simulink model "RTR_2st"  (R2020a)
settings: Solver=ode45  StartTime=0.0  StopTime=T  RelTol=1e-8
values from neighbouring files (symbols this model uses):
  g = 9.81    [TestingIkRTR.m]    (also in TestingScript.m; TestingScriptRTR.m)
  Kd1 = Kp1/10    (= 100)    [TestingIkRTR.m]    (also in TestingScript.m; TestingScriptRTR.m)
  Kp1 = 1000    [TestingIkRTR.m]    (also in TestingScript.m; TestingScriptRTR.m)
  l2 = 0.3    [TestingIkRTR.m]    (also in TestingScriptRTR.m)
  l3 = 0.2    [TestingIkRTR.m]    (also in TestingScriptRTR.m)
  m2 = 20    [TestingIkRTR.m]    (also in TestingScriptRTR.m)
  m3 = 20    [TestingIkRTR.m]    (also in TestingScriptRTR.m)
  O4 = 0.77    [TestingScript.m]
settings Model: Creator=ja  LastModifiedBy=ja

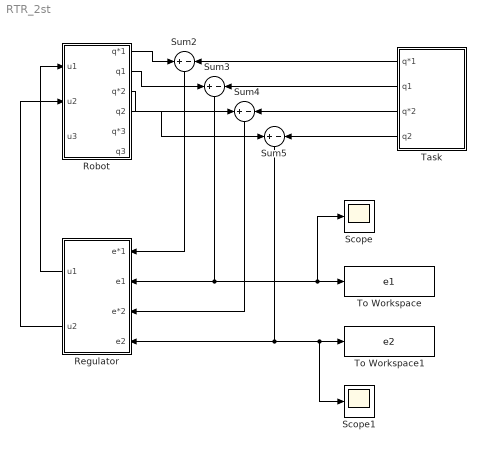
== system RTR_2st ==
  Regulator : Subsystem
  Robot : Subsystem
  Scope : Scope
  Scope1 : Scope
  Sum{2..5} (4 alike) : Sum  Inputs=+-
  Task : Subsystem
  To Workspace : ToWorkspace  VariableName=e1  SampleTime=-1
  To Workspace1 : ToWorkspace  VariableName=e2  SampleTime=-1
  wires:
  Sum4/1 -> Regulator/3(e*2)
  Sum3/1 -> Regulator/2(e1), Scope/1, To Workspace/1
  Sum2/1 -> Regulator/1(e*1)
  Robot/3(q*2) -> Sum4/1
  Robot/4(q2) -> Sum5/1
  Task/1(q*1) -> Sum2/2
  Sum5/1 -> Regulator/4(e2), Scope1/1, To Workspace1/1
  Robot/2(q1) -> Sum3/1
  Task/2(q1) -> Sum3/2
  Regulator/1(" u1") -> Robot/1(u1)
  Task/4(q2) -> Sum5/2
  Regulator/2(u2) -> Robot/2(u2)
  Robot/1(q*1) -> Sum2/1
  Task/3(q*2) -> Sum4/2

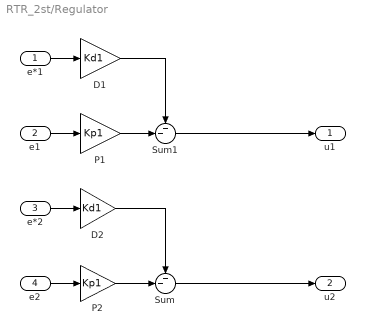
== system RTR_2st/Regulator ==
  e*1 : Inport
  e1 : Inport  Port=2
  e*2 : Inport  Port=3
  e2 : Inport  Port=4
  D1 : Gain  Gain=Kd1
  D2 : Gain  Gain=Kd1
  P1 : Gain  Gain=Kp1
  P2 : Gain  Gain=Kp1
  Sum : Sum  Inputs=--|
  Sum1 : Sum  Inputs=--|
  " u1" : Outport
  u2 : Outport  Port=2
  wires:
  e2/1 -> P2/1
  Sum/1 -> u2/1
  e*2/1 -> D2/1
  e1/1 -> P1/1
  Sum1/1 -> " u1"/1
  e*1/1 -> D1/1
  D1/1 -> Sum1/1
  P1/1 -> Sum1/2
  D2/1 -> Sum/1
  P2/1 -> Sum/2

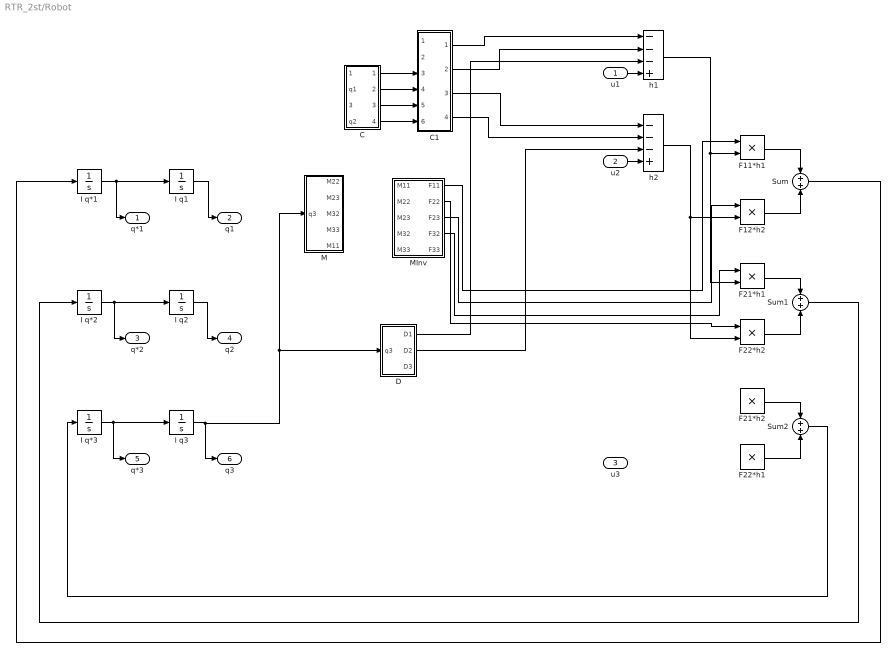
== system RTR_2st/Robot ==
  u1 : Inport
  u2 : Inport  Port=2
  u3 : Inport  Port=3
  C : Subsystem
  C1 : Subsystem
  D : Subsystem
  F11*h1 : Product
  F12*h2 : Product
  F21*h1 : Product
  F21*h2 : Product
  F22*h1 : Product
  F22*h2 : Product
  I q*1 : Integrator
  I q*2 : Integrator
  I q*3 : Integrator
  I q1 : Integrator
  I q2 : Integrator
  I q3 : Integrator
  M : Subsystem
  MInv : MATLAB Function  TreatAsAtomicUnit=on
  Sum : Sum
  Sum1 : Sum
  Sum2 : Sum
  h1 : Sum  Inputs=---+
  h2 : Sum  Inputs=---+
  q*1 : Outport
  q1 : Outport  Port=2
  q*2 : Outport  Port=3
  q2 : Outport  Port=4
  q*3 : Outport  Port=5
  q3 : Outport  Port=6
  wires:
  I q2/1 -> q2/1
  Sum/1 -> I q*1/1
  MInv/1(F11) -> F11*h1/1
  D/1(D1) -> h1/3
  I q*1/1 -> q*1/1, I q1/1
  Sum1/1 -> I q*2/1
  I q1/1 -> q1/1
  F22*h2/1 -> Sum1/2
  F11*h1/1 -> Sum/1
  I q*2/1 -> q*2/1, I q2/1
  MInv/2(F22) -> F22*h2/1
  F12*h2/1 -> Sum/2
  D/2(D2) -> h2/3
  h2/1 -> F12*h2/2, F22*h2/2
  F21*h1/1 -> Sum1/1
  u2/1 -> h2/4
  MInv/3(F23) -> F12*h2/1
  h1/1 -> F21*h1/2, F11*h1/2
  u1/1 -> h1/4
  C/1(C11) -> C1/3(C11)
  C/2(C12) -> C1/4(C12)
  C/3(C21) -> C1/5(C21)
  C/4(C22) -> C1/6(C22)
  C1/4(Out4) -> h2/2
  C1/3(Out3) -> h2/1
  C1/1(Out1) -> h1/1
  C1/2(Out2) -> h1/2
  MInv/4(F32) -> F21*h1/1
  F21*h2/1 -> Sum2/1
  F22*h1/1 -> Sum2/2
  Sum2/1 -> I q*3/1
  I q*3/1 -> q*3/1, I q3/1
  I q3/1 -> M/1(q3), D/1(q3), q3/1

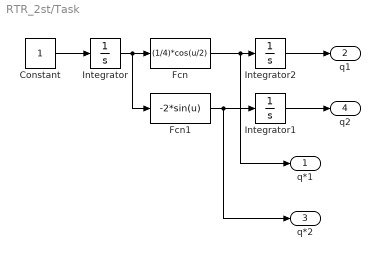
== system RTR_2st/Task ==
  Constant : Constant
  Fcn : Fcn  Expr=(1/4)*cos(u/2)
  Fcn1 : Fcn  Expr=-2*sin(u)
  Integrator : Integrator
  Integrator1 : Integrator  InitialCondition=2
  Integrator2 : Integrator
  q*1 : Outport
  q1 : Outport  Port=2
  q*2 : Outport  Port=3
  q2 : Outport  Port=4
  wires:
  Constant/1 -> Integrator/1
  Integrator/1 -> Fcn1/1, Fcn/1
  Fcn/1 -> q*1/1, Integrator2/1
  Fcn1/1 -> q*2/1, Integrator1/1
  Integrator2/1 -> q1/1
  Integrator1/1 -> q2/1

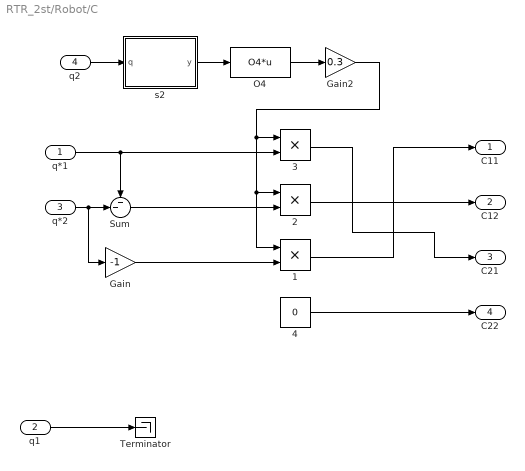
== system RTR_2st/Robot/C ==
  q*1 : Inport
  q1 : Inport  Port=2
  q*2 : Inport  Port=3
  q2 : Inport  Port=4
  1 : Product
  2 : Product
  3 : Product
  4 : Constant  Value=0
  Gain : Gain  Gain=-1
  Gain2 : Gain  Gain=0.3
  O4 : Fcn  Expr=O4*u
  Sum : Sum  Inputs=--|
  Terminator : Terminator
  s2 : MATLAB Function  TreatAsAtomicUnit=on
  C11 : Outport
  C12 : Outport  Port=2
  C21 : Outport  Port=3
  C22 : Outport  Port=4
  wires:
  q*2/1 -> Gain/1, Sum/2
  q2/1 -> s2/1(q)
  q*1/1 -> 3/2, Sum/1
  s2/1(y) -> O4/1
  O4/1 -> Gain2/1
  Sum/1 -> 2/2
  Gain/1 -> 1/2
  Gain2/1 -> 1/1, 2/1, 3/1
  4/1 -> C22/1
  1/1 -> C11/1
  3/1 -> C21/1
  2/1 -> C12/1
  q1/1 -> Terminator/1

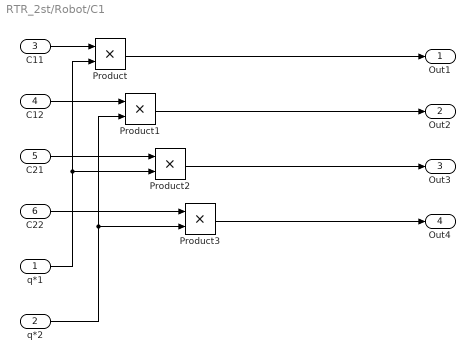
== system RTR_2st/Robot/C1 ==
  q*1 : Inport
  q*2 : Inport  Port=2
  C11 : Inport  Port=3
  C12 : Inport  Port=4
  C21 : Inport  Port=5
  C22 : Inport  Port=6
  Product{,1..3} (4 alike) : Product
  Out1 : Outport
  Out2 : Outport  Port=2
  Out3 : Outport  Port=3
  Out4 : Outport  Port=4
  wires:
  C11/1 -> Product/1
  C12/1 -> Product1/1
  C21/1 -> Product2/1
  C22/1 -> Product3/1
  q*1/1 -> Product2/2, Product/2
  q*2/1 -> Product3/2, Product1/2
  Product3/1 -> Out4/1
  Product2/1 -> Out3/1
  Product1/1 -> Out2/1
  Product/1 -> Out1/1

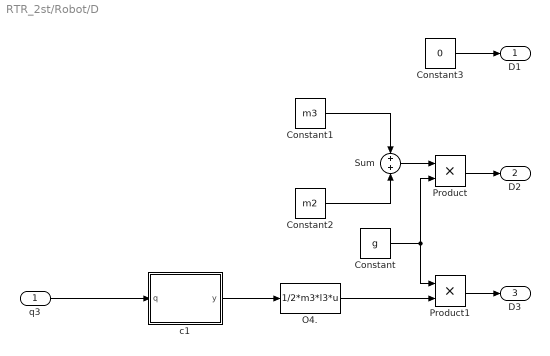
== system RTR_2st/Robot/D ==
  q3 : Inport
  Constant : Constant  Value=g
  Constant1 : Constant  Value=m3
  Constant2 : Constant  Value=m2
  Constant3 : Constant  Value=0
  O4. : Fcn  Expr=1/2*m3*l3*u
  Product : Product
  Product1 : Product
  Sum : Sum
  c1 : MATLAB Function  TreatAsAtomicUnit=on
  D1 : Outport
  D2 : Outport  Port=2
  D3 : Outport  Port=3
  wires:
  c1/1(y) -> O4./1
  Sum/1 -> Product/1
  Constant/1 -> Product/2, Product1/1
  O4./1 -> Product1/2
  Constant2/1 -> Sum/2
  Constant1/1 -> Sum/1
  q3/1 -> c1/1(q)
  Product/1 -> D2/1
  Product1/1 -> D3/1
  Constant3/1 -> D1/1

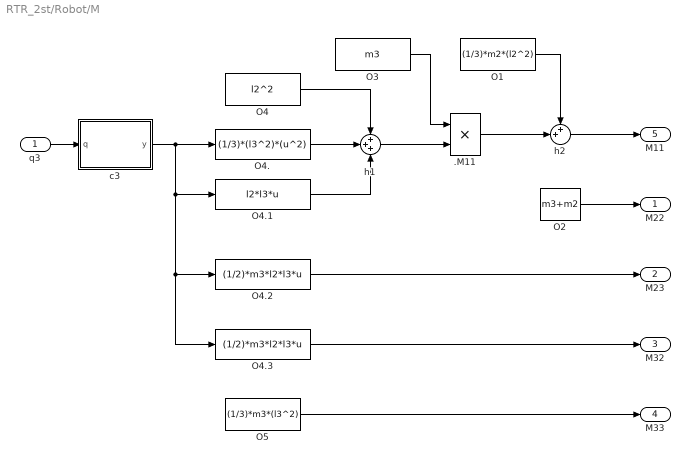
== system RTR_2st/Robot/M ==
  q3 : Inport
  .M11 : Product
  O1 : Constant  Value=(1/3)*m2*(l2^2)
  O2 : Constant  Value=m3+m2
  O3 : Constant  Value=m3
  O4 : Constant  Value=l2^2
  O4. : Fcn  Expr=(1/3)*(l3^2)*(u^2)
  O4.1 : Fcn  Expr=l2*l3*u
  O4.2 : Fcn  Expr=(1/2)*m3*l2*l3*u
  O4.3 : Fcn  Expr=(1/2)*m3*l2*l3*u
  O5 : Constant  Value=(1/3)*m3*(l3^2)
  c3 : MATLAB Function  TreatAsAtomicUnit=on
  h1 : Sum  Inputs=+++
  h2 : Sum  Inputs=++|
  M22 : Outport
  M23 : Outport  Port=2
  M32 : Outport  Port=3
  M33 : Outport  Port=4
  M11 : Outport  Port=5
  wires:
  O1/1 -> h2/1
  O4.1/1 -> h1/3
  O3/1 -> .M11/1
  h1/1 -> .M11/2
  .M11/1 -> h2/2
  O4/1 -> h1/1
  O4./1 -> h1/2
  h2/1 -> M11/1
  O2/1 -> M22/1
  O4.2/1 -> M23/1
  c3/1(y) -> O4./1, O4.3/1, O4.2/1, O4.1/1
  q3/1 -> c3/1(q)
  O5/1 -> M33/1
  O4.3/1 -> M32/1

== matlab function RTR_2st/Robot/M/c3 ==
  data: q input; y output
function y = c(q)

y = cos(q);

== matlab function RTR_2st/Robot/D/c1 ==
  data: q input; y output
function y = c(q)

y = cos(q);

== matlab function RTR_2st/Robot/C/s2 ==
  data: q input; y output
function y = s(q)

y = sin(q);

== matlab function RTR_2st/Robot/MInv ==
  data: M11 input; M22 input; F11 output; F22 output; M23 input; M32 input; F23 output; F32 output; M33 input; F33 output
function [F11, F22, F23, F32, F33] = c(M11, M22, M23, M32, M33)

M = [M11 0 0; 0 M22 M23; 0 M32 M33];
F = inv(M);

F11 = F(1);
F22 = F(5);
F23 = F(6);
F32 = F(8);
F33 = F(9);
